simulink model "BrakingSystemPlant"  (Simulink 8.5)
settings: Solver=ode45  StartTime=0.0  StopTime=25  RelTol=1e-3
values from neighbouring files (symbols this model uses):
  brakegapNom = 4    [simParameters.m]
  mpod = 360.    (= 360)    [simParameters.m]
  rho = P/(R*T)    (= 0.0102419279583)    [simParameters.m]
  xdot3 = xdot(n)    [Trajectory.m]
  z_nom = 0.016    [simParameters.m]
settings Model: Creator=MrPiccolo  LastModifiedBy=Krillin
settings DataIOCC: SignalLoggingSaveFormat=Dataset
settings OptimizationCC: ExpressionDepthLimit=128
settings DebuggingCC: UnderspecifiedInitializationDetection=Simplified  MergeDetectMultiDrivingBlocksExec=error  FcnCallInpInsideContextMsg=EnableAllAsError  StateNameClashWarn=none
settings GRTTargetCC: CombineOutputUpdateFcns=on  GRTInterface=off

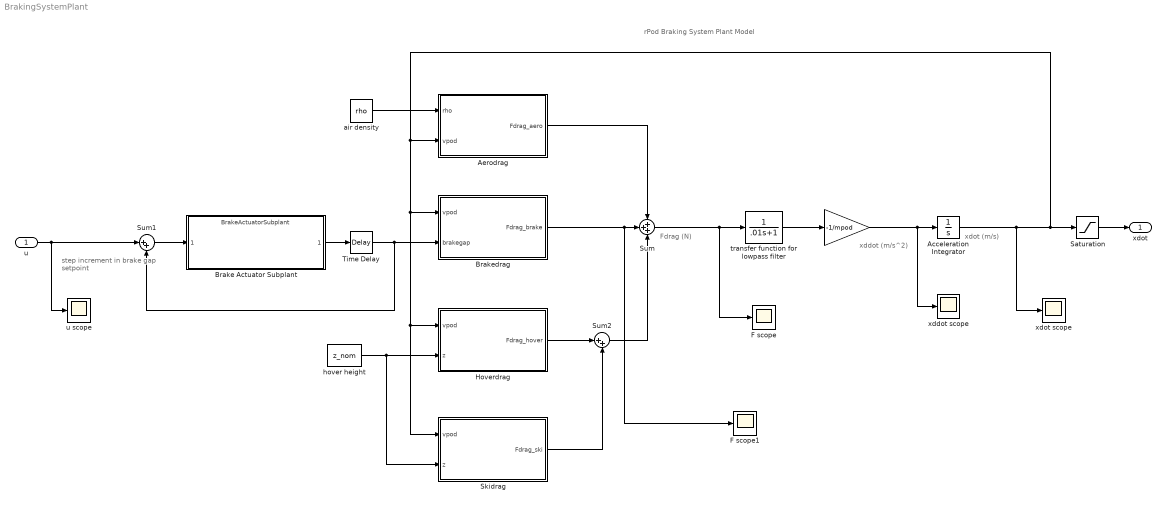
== system BrakingSystemPlant ==
  note: Fdrag (N)
  note: xddot (m/s^2)
  note: xdot (m/s)
  note: rPod Braking System
      | Plant Model
  note: step increment in
      | brake gap setpoint
  u : Inport
  " " : Gain  Gain=-1/mpod
  Acceleration Integrator : Integrator  InitialCondition=xdot3  LimitOutput=on  LowerSaturationLimit=0
  Aerodrag : MATLAB Function  TreatAsAtomicUnit=on
  Brake Actuator Subplant : ModelReference  ModelNameDialog=BrakeActuatorSubplant.mdl  SimulationMode=Normal  ModelReferenceVersion=1.130  CopyOfModelName=BrakeActuatorSubplant.mdl  DefaultDataLogging=on
  Brakedrag : MATLAB Function  TreatAsAtomicUnit=on
  F scope : Scope
      settings: SaveName=ScopeData5
  F scope1 : Scope
  Hoverdrag : MATLAB Function  TreatAsAtomicUnit=on
  Saturation : Saturate  UpperLimit=300  LowerLimit=0
  Skidrag : MATLAB Function  TreatAsAtomicUnit=on
  Sum : Sum  Inputs=+++
  Sum1 : Sum  Inputs=|++
  Sum2 : Sum  Inputs=|++
  Time Delay : TransportDelay  DelayTime=.05  InitialOutput=brakegapNom
  air density : Constant  Value=rho
  hover height : Constant  Value=z_nom
  transfer function for lowpass filter : TransferFcn  Denominator=[.01 1]
  u scope : Scope
      settings: YMin=2.09908  YMax=25.3146
  xddot scope : Scope
      settings: SaveName=ScopeData4
  xdot scope : Scope
      settings: TimeRange=40  YMin=12.1094  YMax=20.7376  SaveName=ScopeData2
  xdot : Outport
  wires:
  " "/1 -> xddot scope/1, Acceleration Integrator/1
  Brake Actuator Subplant/1 -> Time Delay/1
  Acceleration Integrator/1 -> xdot scope/1, Skidrag/1(vpod), Hoverdrag/1(vpod), Brakedrag/1(vpod), Aerodrag/2(vpod), Saturation/1
  u/1 -> Sum1/1, u scope/1
  Saturation/1 -> xdot/1
  Time Delay/1 -> Brakedrag/2(brakegap), Sum1/2
  Brakedrag/1(Fdrag_brake) -> F scope1/1, Sum/2
  air density/1 -> Aerodrag/1(rho)
  Aerodrag/1(Fdrag_aero) -> Sum/1
  transfer function for lowpass filter/1 -> " "/1
  Sum1/1 -> Brake Actuator Subplant/1
  Sum/1 -> F scope/1, transfer function for lowpass filter/1
  hover height/1 -> Hoverdrag/2(z), Skidrag/2(z)
  Hoverdrag/1(Fdrag_hover) -> Sum2/1
  Sum2/1 -> Sum/3
  Skidrag/1(Fdrag_ski) -> Sum2/2

== matlab function Aerodrag ==
  data: rho input double; vpod input double; Fdrag_aero output double
function Fdrag_aero = fcn(rho, vpod)
%#codegen

Fdrag_aero = Fdrag.aero(vpod,rho);

== matlab function Brakedrag ==
  data: vpod input double; brakegap input double; Fdrag_brake output double
function Fdrag_brake = fcn(vpod, brakegap)
%#codegen

Fdrag_brake = Fdrag.brake(vpod, brakegap);

== matlab function Hoverdrag ==
  data: vpod input double; z input double; Fdrag_hover output double
function Fdrag_hover = fcn(vpod, z)
%#codegen

Fdrag_hover = Fdrag.hover(vpod, z);

== matlab function Skidrag ==
  data: vpod input double; z input double; Fdrag_ski output double
function Fdrag_ski = fcn(vpod,z)
%#codegen

Fdrag_ski = Fdrag.ski(vpod,z);
